simulink model "Rot3DOF"  (R2013b)
settings: Solver=ode45  StartTime=0.0  StopTime=10.0  RelTol=1e-3
settings Model: Creator=rskjetne  LastModifiedBy=rskjetne

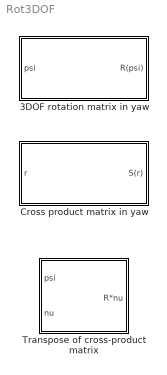
== system Rot3DOF ==
  3DOF rotation matrix in yaw : Subsystem
      mask help:
      | 3DOF rotation matrix in yaw
      | where
      |
      | input 1:    psi
      | output 1:  R(psi) - matrix dim 3x3
      |
      | % Roger Skjetne - 08.03.2014
      mask Display:
      | port_label('output', 1, 'R(psi)')
      | port_label('input', 1, 'psi')
  Cross product matrix in yaw : Subsystem
      mask help:
      | 3DOF cross product matrix S(r) in yaw
      | where
      |
      | input 1:    r
      | output 1:  S(r) - matrix dim 3x3
      |
      | % Roger Skjetne - 08.03.2014
      mask Display:
      | port_label('output', 1, 'S(r)')
      | port_label('input', 1, 'r')
  Transpose of cross-product matrix : Subsystem
      mask help:
      | y = transpose(S(r)) * x
      |
      | where
      |
      | input 1:    r
      | input 2:    x - vector dim 3
      | output 1:  y - vector dim 3
      mask Display:
      | port_label('output', 1, 'tr(S(r))*x')
      | port_label('input', 1, 'r')
      | port_label('input', 2, 'x')

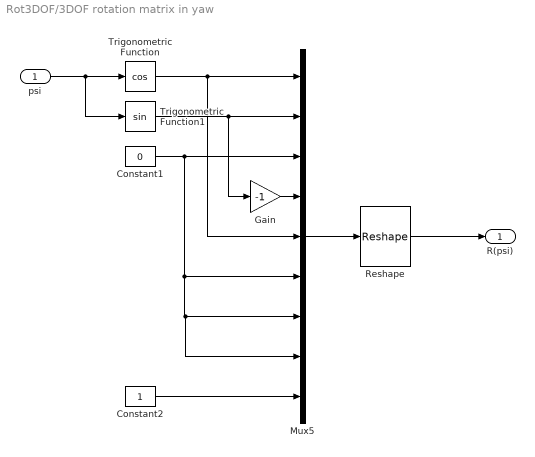
== system Rot3DOF/3DOF rotation matrix in yaw ==
  psi : Inport
  Constant1 : Constant  Value=0
  Constant2 : Constant
  Gain : Gain  Gain=-1
  Mux5 : Mux  Inputs=9
  Reshape : Reshape  OutputDimensionality=Customize  OutputDimensions=[3,3]
  Trigonometric Function : Trigonometry  Operator=cos
  Trigonometric Function1 : Trigonometry
  R(psi) : Outport
  wires:
  Mux5/1 -> Reshape/1
  psi/1 -> Trigonometric Function1/1, Trigonometric Function/1
  Trigonometric Function/1 -> Mux5/5, Mux5/1
  Trigonometric Function1/1 -> Gain/1, Mux5/2
  Constant1/1 -> Mux5/8, Mux5/7, Mux5/6, Mux5/3
  Reshape/1 -> R(psi)/1
  Gain/1 -> Mux5/4
  Constant2/1 -> Mux5/9

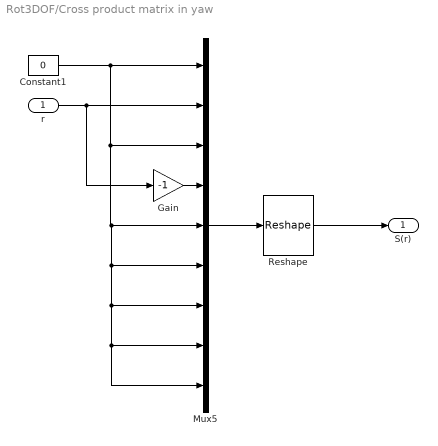
== system Rot3DOF/Cross product matrix in yaw ==
  r : Inport
  Constant1 : Constant  Value=0
  Gain : Gain  Gain=-1
  Mux5 : Mux  Inputs=9
  Reshape : Reshape  OutputDimensionality=Customize  OutputDimensions=[3,3]
  S(r) : Outport
  wires:
  Gain/1 -> Mux5/4
  Reshape/1 -> S(r)/1
  Mux5/1 -> Reshape/1
  Constant1/1 -> Mux5/9, Mux5/8, Mux5/7, Mux5/6, Mux5/5, Mux5/3, Mux5/1
  r/1 -> Gain/1, Mux5/2

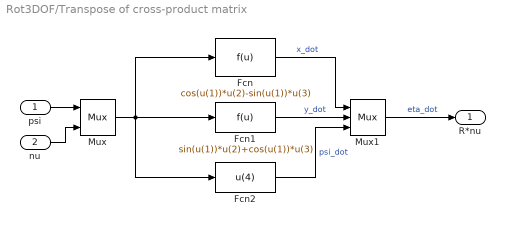
== system Rot3DOF/Transpose of cross-product matrix ==
  psi : Inport
  nu : Inport  Port=2
  Fcn : Fcn  Expr=cos(u(1))*u(2)-sin(u(1))*u(3)
  Fcn1 : Fcn  Expr=sin(u(1))*u(2)+cos(u(1))*u(3)
  Fcn2 : Fcn  Expr=u(4)
  Mux : Mux  Inputs=2
  Mux1 : Mux  Inputs=3
  R*nu : Outport
  wires:
  nu/1 -> Mux/2
  psi/1 -> Mux/1
  Mux1/1 -> R*nu/1  "eta_dot"
  Fcn2/1 -> Mux1/3  "psi_dot"
  Fcn1/1 -> Mux1/2  "y_dot"
  Fcn/1 -> Mux1/1  "x_dot"
  Mux/1 -> Fcn/1, Fcn1/1, Fcn2/1
